simulink model "L07_Ex3"  (R2020b)
settings: Solver=VariableStepAuto  StartTime=0.0  StopTime=10.0  RelTol=1e-3
settings Model: Creator=Nic  LastModifiedBy=Nic

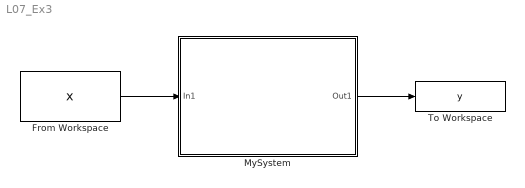
== system L07_Ex3 ==
  From Workspace : FromWorkspace  VariableName=x  SampleTime=-1
  MySystem : Subsystem
  To Workspace : ToWorkspace  VariableName=y  SampleTime=-1
  wires:
  From Workspace/1 -> MySystem/1(In1)
  MySystem/1(Out1) -> To Workspace/1

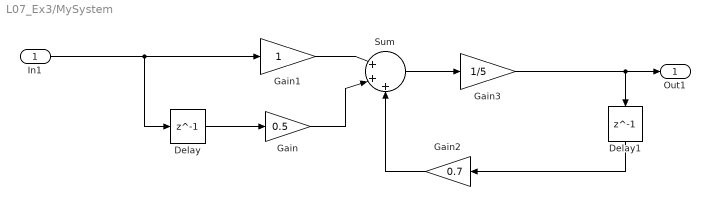
== system L07_Ex3/MySystem ==
  In1 : Inport
  Delay : Delay  DelayLength=1  InitialCondition=0
  Delay1 : Delay  DelayLength=1  InitialCondition=0
  Gain : Gain  Gain=0.5
  Gain1 : Gain
  Gain2 : Gain  Gain=0.7
  Gain3 : Gain  Gain=1/5
  Sum : Sum  Inputs=|+++
  Out1 : Outport
  wires:
  Delay1/1 -> Gain2/1
  Gain1/1 -> Sum/1
  Gain2/1 -> Sum/3
  Delay/1 -> Gain/1
  Gain/1 -> Sum/2
  Sum/1 -> Gain3/1
  In1/1 -> Delay/1, Gain1/1
  Gain3/1 -> Out1/1, Delay1/1
